simulink model "CirclwRobotModel"  (R2023b)
settings: Solver=VariableStepAuto  StartTime=0.0  StopTime=10.0  RelTol=1e-3
InitFcn:
  | r = 0.1; % радиус колеса
  | a = 0.2;
settings Model: Creator=ACER1  LastModifiedBy=ACER1

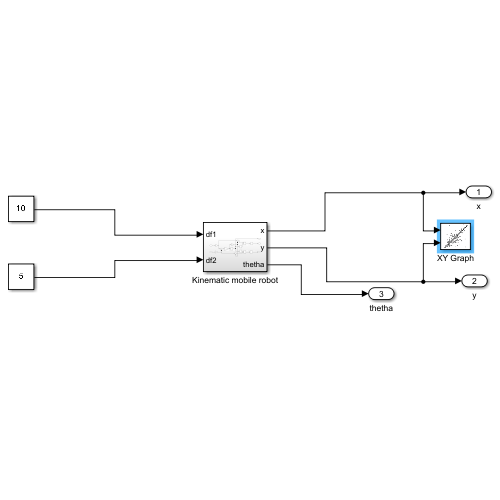
[thumbnail: Simulink's stored preview of the top-level diagram]
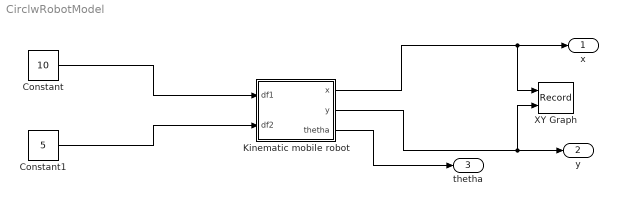
== system CirclwRobotModel ==
  Constant : Constant  Value=10
  Constant1 : Constant  Value=5
  Kinematic mobile robot : Subsystem
  XY Graph : Record  FileSettingsInternal="{\"entries\":[{\"content\":{\"excelSettings\":{\"content\":{},\"type\":\"Streamout.ExcelSettings\"}},\"type\":\"Streamout.FileSettingStorage\",\"uuid\":\"\"}],\"packageUris\":[\"http:\\/\\/schema.mathworks.com\\/mf0\\/streamout_blocks\\/R2020a\"],\"version\":\"1.0\"}"  Layout=[1 1]  SignalsInternal="{\"entries\":[{\"content\":{\"signals\":[{\"content\":{\"blockPath\":[],\"dimensions\":[1],\"domain\":\"\",\"lineColor\":\"#a2142f\",\"plots\":[1],\"port\":1,\"sid\":[\"\"],\"signalID\":249,\"signalName\":\"Kinematic mobile robot:1\"},\"type\":\"RecordBlkView.Signal\",\"uuid\":\"\"},{\"content\":{\"blockPath\":[],\"dimensions\":[1],\"domain\":\"\",\"lineColor\":\"#139fff\",\"plots\":[1],\"port\":2,\"sid\":[\"\"],\"signalID\":253,\"signalName\":\"Kinematic mobile robot:2\"},\"type\":\"RecordBlkView.Signal\",\"uuid\":\"\"}]},\"type\":\"RecordBlkView.InputSignals\",\"uuid\":\"\"}],\"packageUris\":[\"http:\\/\\/schema.mathworks.com\\/mf0\\/streamout_blocks\\/R2020a\"],\"version\":\"1.0\"}"  VisualizationBindings="{\"xyplotplugin\":{\"info\":[{\"series\":[{\"bindingParametersList\":[{\"parameter\":\"X-Axis\",\"signalID\":249,\"signalName\":\"Kinematic mobile robot:1\"},{\"parameter\":\"Y-Axis\",\"signalID\":253,\"signalName\":\"Kinematic mobile robot:2\"}],\"seriesID\":57612}],\"subplotID\":1}]}}"  CompatibilityTag=XY
  x : Outport
  y : Outport  Port=2
  thetha : Outport  Port=3
  wires:
  Constant/1 -> Kinematic mobile robot/1(df1)
  Constant1/1 -> Kinematic mobile robot/2(df2)
  Kinematic mobile robot/1(x) -> XY Graph/1, x/1
  Kinematic mobile robot/3(thetha) -> thetha/1
  Kinematic mobile robot/2(y) -> XY Graph/2, y/1

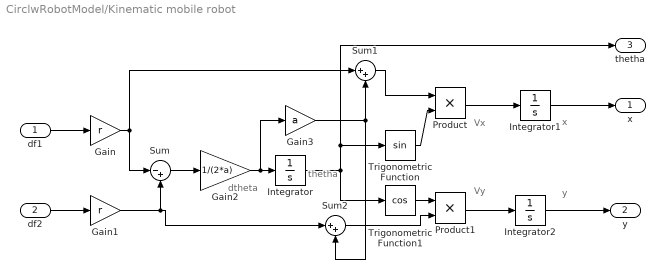
== system CirclwRobotModel/Kinematic mobile robot ==
  note: thetha
  note: y
  note: x
  note: Vy
  note: Vx
  note: dtheta
  df1 : Inport
  df2 : Inport  Port=2
  Gain : Gain  Gain=r
  Gain1 : Gain  Gain=r
  Gain2 : Gain  Gain=1/(2*a)
  Gain3 : Gain  Gain=a
  Integrator : Integrator
  Integrator1 : Integrator
  Integrator2 : Integrator
  Product : Product
  Product1 : Product
  Sum : Sum  Inputs=|-+
  Sum1 : Sum  Inputs=|++
  Sum2 : Sum  Inputs=|++
  Trigonometric Function : Trigonometry
  Trigonometric Function1 : Trigonometry  Operator=cos
  x : Outport
  y : Outport  Port=2
  thetha : Outport  Port=3
  wires:
  Gain3/1 -> Sum2/2, Sum1/2
  df2/1 -> Gain1/1
  Gain1/1 -> Sum2/1, Sum/2
  Integrator/1 -> Trigonometric Function1/1, thetha/1, Trigonometric Function/1
  df1/1 -> Gain/1
  Gain2/1 -> Integrator/1, Gain3/1
  Gain/1 -> Sum1/1, Sum/1
  Sum2/1 -> Product1/2
  Trigonometric Function1/1 -> Product1/1
  Product1/1 -> Integrator2/1
  Trigonometric Function/1 -> Product/2
  Sum/1 -> Gain2/1
  Integrator2/1 -> y/1
  Product/1 -> Integrator1/1
  Sum1/1 -> Product/1
  Integrator1/1 -> x/1
